simulink model "parafoil_model"  (R2022a)
settings: Solver=VariableStepAuto  StartTime=0.0  StopTime=200  MaxStep=0.01  RelTol=1e-3
undefined symbols (not defined in the file or in its folder): controller
settings Model: Creator=12230  LastModifiedBy=12230
settings DataIOCC: ReturnWorkspaceOutputs=off

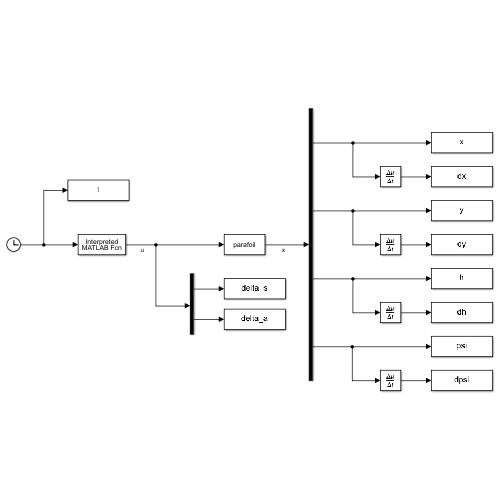
[thumbnail: Simulink's stored preview of the top-level diagram]
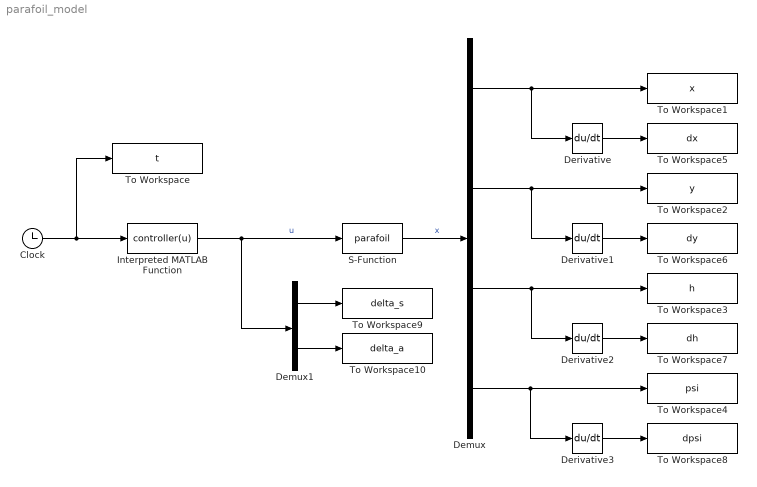
== system parafoil_model ==
  Clock : Clock
  Demux : Demux
  Demux1 : Demux  Outputs=2
  Derivative{,1..3} (4 alike) : Derivative
  Interpreted MATLAB Function : MATLABFcn  MATLABFcn=controller(u)
  S-Function : S-Function  FunctionName=parafoil  SFunctionDeploymentMode=off  EnableBusSupport=off
  To Workspace : ToWorkspace  VariableName=t  SampleTime=-1
  To Workspace1 : ToWorkspace  VariableName=x  SampleTime=-1
  To Workspace10 : ToWorkspace  VariableName=delta_a  SampleTime=-1
  To Workspace2 : ToWorkspace  VariableName=y  SampleTime=-1
  To Workspace3 : ToWorkspace  VariableName=h  SampleTime=-1
  To Workspace4 : ToWorkspace  VariableName=psi  SampleTime=-1
  To Workspace5 : ToWorkspace  VariableName=dx  SampleTime=-1
  To Workspace6 : ToWorkspace  VariableName=dy  SampleTime=-1
  To Workspace7 : ToWorkspace  VariableName=dh  SampleTime=-1
  To Workspace8 : ToWorkspace  VariableName=dpsi  SampleTime=-1
  To Workspace9 : ToWorkspace  VariableName=delta_s  SampleTime=-1
  wires:
  Clock/1 -> Interpreted MATLAB Function/1, To Workspace/1
  Interpreted MATLAB Function/1 -> Demux1/1, S-Function/1  "u"
  Demux/1 -> Derivative/1, To Workspace1/1
  S-Function/1 -> Demux/1  "x"
  Derivative/1 -> To Workspace5/1
  Derivative1/1 -> To Workspace6/1
  Demux/2 -> Derivative1/1, To Workspace2/1
  Derivative2/1 -> To Workspace7/1
  Demux/3 -> Derivative2/1, To Workspace3/1
  Derivative3/1 -> To Workspace8/1
  Demux/4 -> Derivative3/1, To Workspace4/1
  Demux1/1 -> To Workspace9/1
  Demux1/2 -> To Workspace10/1
